simulink model "Ecuacion_Diferencial_Codigo_Ejercicio_6"  (R2017b)
settings: Solver=VariableStepAuto  StartTime=0.0  StopTime=10.0  RelTol=1e-3
settings Model: Creator=Elmer  LastModifiedBy=Elmer

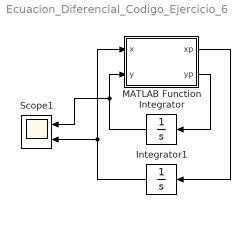
== system Ecuacion_Diferencial_Codigo_Ejercicio_6 ==
  Integrator : Integrator  InitialCondition=0.5
  Integrator1 : Integrator  InitialCondition=0.5
  MATLAB Function : MATLAB Function  TreatAsAtomicUnit=on
  Scope1 : Scope  NumInputPorts=2
  wires:
  MATLAB Function/1(xp) -> Integrator1/1
  Integrator1/1 -> Scope1/2, MATLAB Function/1(x)
  MATLAB Function/2(yp) -> Integrator/1
  Integrator/1 -> Scope1/1, MATLAB Function/2(y)

== matlab function Ecuacion_Diferencial_Codigo_Ejercicio_6/MATLAB Function ==
  data: x input; y input; xp output; yp output
function [xp,yp]= fcn(x,y)
xp=3*x + 4*y;
yp=5*x - 7*y;
